simulink model "Protection"  (R2023b)
settings: Solver=FixedStepAuto  StartTime=0.0  StopTime=2  RelTol=1e-3
InitFcn:
  | Ts_Control=100e-6;
  | fs=50000;
  | Ts=1/fs/10;
  | Ts_Power=Ts;
  | Ts_control=5*Ts;
  | wnom=314.16;
  | Lf=5e-3;
  | Rf=0.1;
  | Cf=50e-6;
  | 
  | 
  | % choosing crossover frequency
  | fc=(1/10)*fs;
  | wc=2*pi*fc;
  | Ti=1/wc;
  | Kpc=Lf/Ti;
  | 
  | Kic=Rf/Ti;
  | 
  | x=[837.555 8.2389 0.057896 268.1361 0.74685 242.918 0.062838 291.0935]
  | 
  | 
  | Kvi=x(1);Kvp=x(2);Kcp=x(3);Kci=x(4);
  | Kvpb=x(5);Kvib=x(6);Kcpb=x(7);Kcib=x(8);
  | 
  | 
  | x1=[0.202905850069502  0.158544693742674   0.10408       75.97091  837.555350377473 8.2389271001531  0.10408       75.97091];
  | 
  | Kvif=x1(1);Kvpf=x1(2);Kcpf=x1(3);Kcif=x1(4);
  | Kvim=x1(5);Kvpm=x1(6);Kcpm=x1(7);Kcim=x1(8);
undefined symbols (not defined in the file): D1, Delta, Hydride, Metal, Nickel, sigbuilder_block
libraries: spsSeriesRLCBranchLib x52, spsVoltageMeasurementLib x22, powerlib_extras x18, spsCurrentMeasurementLib x13, spsIdealSwitchLib x12, simulink x8, slpidlib x7, spsGroundLib x6, spsBreakerLib x5, spsDiodeLib x4, spsIGBTLib x4, spsThreePhaseVIMeasurementLib x4
(part 1 of 2)
settings Model: Creator=shiva  LastModifiedBy=vnougain
settings SolverCC: AlgebraicLoopSolver=TrustRegion
settings DataIOCC: LimitDataPoints=on  SaveOutput=off  SaveTime=off  ReturnWorkspaceOutputs=off
settings OptimizationCC: EfficientMapNaN2IntZero=off  LifeSpan=inf
settings DebuggingCC: UnconnectedInputMsg=warning  UnconnectedOutputMsg=warning  UnconnectedLineMsg=warning  AllowSymbolicDim=off  SFUnexpectedBacktrackingDiag=warning  SFNoUnconditionalDefaultTransitionDiag=warning  SFExecutionAtInitializationDiag=none  ArithmeticOperatorsInVariantConditions=warning
settings HardwareCC: ProdBitPerChar=16  ProdBitPerInt=16  ProdBitPerPointer=32  ProdBitPerSizeT=32  ProdBitPerPtrDiffT=32  ProdLargestAtomicInteger=Integer  ProdLargestAtomicFloat=None  ProdWordSize=16  ProdHWDeviceType=Texas Instruments->C2000  TargetBitPerPointer=64  TargetBitPerSizeT=64  TargetBitPerPtrDiffT=64  TargetLongLongMode=on  TargetIntDivRoundTo=Zero  TargetEndianess=LittleEndian  TargetWordSize=64  TargetHWDeviceType=MATLAB Host  ProdEqTarget=off
settings ModelReferenceCC: EnableRefExpFcnMdlSchedulingChecks=on  PropagateSignalLabelsOutOfModel=off
settings SFSimCC: SimUseLocalCustomCode=off  CustomCodeUndefinedFunction=UseInterfaceOnly
settings RTWCC: RTWUseLocalCustomCode=off
settings CodeAppCC: MaxIdLength=128  StateflowObjectComments=on
settings GRTTargetCC: TargetLangStandard=C89/C90 (ANSI)  CombineOutputUpdateFcns=off  GRTInterface=on
settings ConfigComp: CovMetricSettings=dw  CovSaveCumulativeToWorkspaceVar=on  CovSaveSingleToWorkspaceVar=on  CovExternalEMLEnable=off
settings SimscapeCC: SimscapeNormalizeSystem=off
settings TargetHardwareResources: Description=Target Hardware Resources Component

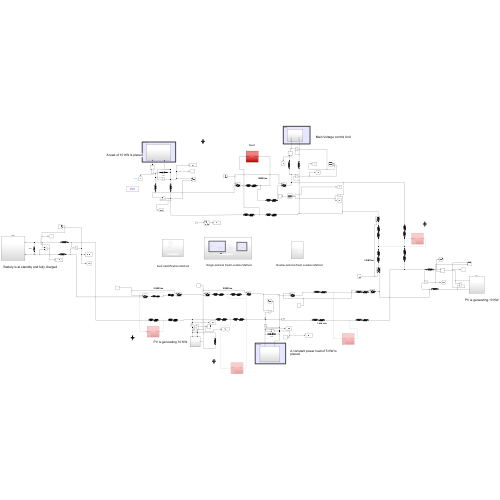
[thumbnail: Simulink's stored preview of the top-level diagram]
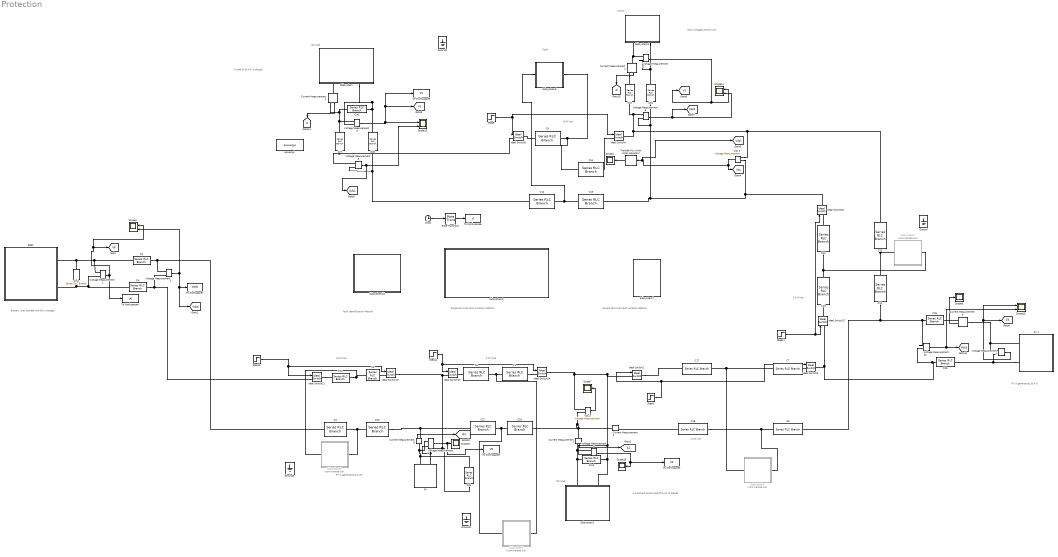
== system Protection ==
  note: Utility
  note: DC load
  note: DC load
  note: 2KM line
  note: 3 KM line
  note: 2 KM line
  note: 1 KM line
  note: 3 KM line
  note: A load of 10 KW is placed
  note: A constant power load of 5 KW is placed
  note: PV is generating 10 KW
  note: Battery is at standby and fully charged
  note: Main Voltage control Unit
  note: Fault
  note: Single-terminal Fault Location Method
  note: Double-terminal Fault Location Method
  note: PV is generating 10 KW
  note: Fault Identification Method
  C{1,6,19,22} (4 alike) : spsSeriesRLCBranchLib/Series RLC Branch  LConnTagsString=__new0  RConnTagsString=__new0  BranchType=RL  Resistance=1*0.3293  Inductance=1*522.026e-6  SetiL0=off  InitialCurrent=0  Capacitance=12000e-06  Setx0=off  InitialVoltage=0  Measurements=None
  C{9..12,23..24} (6 alike) : spsSeriesRLCBranchLib/Series RLC Branch  LConnTagsString=__new0  RConnTagsString=__new0  BranchType=RL  Resistance=0.3293*1.5  Inductance=522.026e-6*1.5  SetiL0=off  InitialCurrent=0  Capacitance=12000e-06  Setx0=off  InitialVoltage=0  Measurements=None
  C13 : spsSeriesRLCBranchLib/Series RLC Branch  LConnTagsString=__new0  RConnTagsString=__new0  BranchType=RL  Resistance=0.3293*0.5  Inductance=522.026e-6*0.5  SetiL0=off  InitialCurrent=0  Capacitance=12000e-06  Setx0=off  InitialVoltage=0  Measurements=None
  C14 : spsSeriesRLCBranchLib/Series RLC Branch  LConnTagsString=__new0  RConnTagsString=__new0  BranchType=RL  Resistance=0.3293*0.5  Inductance=522.026e-6*0.5  SetiL0=off  InitialCurrent=0  Capacitance=12000e-06  Setx0=off  InitialVoltage=0  Measurements=None
  C{15..16,27..28} (4 alike) : spsSeriesRLCBranchLib/Series RLC Branch  LConnTagsString=__new0  RConnTagsString=__new0  BranchType=L  Resistance=1.5*0.3293  Inductance=1e-3  SetiL0=off  InitialCurrent=0  Capacitance=12000e-06  Setx0=off  InitialVoltage=0  Measurements=None
  C{7..8,17..18} (4 alike) : spsSeriesRLCBranchLib/Series RLC Branch  LConnTagsString=__new0  RConnTagsString=__new0  BranchType=RL  Resistance=0.3293/2  Inductance=(522.026e-6)/2  SetiL0=off  InitialCurrent=0  Capacitance=12000e-06  Setx0=off  InitialVoltage=0  Measurements=None
  C2 : spsSeriesRLCBranchLib/Series RLC Branch  LConnTagsString=__new0  RConnTagsString=__new0  BranchType=L  Resistance=1.5*0.3293  Inductance=5e-6  SetiL0=off  InitialCurrent=0  Capacitance=12000e-06  Setx0=off  InitialVoltage=0  Measurements=None
  C{3,5,20..21} (4 alike) : spsSeriesRLCBranchLib/Series RLC Branch  LConnTagsString=__new0  RConnTagsString=__new0  BranchType=RL  Resistance=1.5*0.3293  Inductance=1.5*522.026e-6  SetiL0=off  InitialCurrent=0  Capacitance=12000e-06  Setx0=off  InitialVoltage=0  Measurements=None
  C25 : spsSeriesRLCBranchLib/Series RLC Branch  LConnTagsString=__new0  RConnTagsString=__new0  BranchType=R  Resistance=245  Inductance=1*522.026e-6  SetiL0=off  InitialCurrent=0  Capacitance=12000e-06  Setx0=off  InitialVoltage=0  Measurements=None
  C26 : spsSeriesRLCBranchLib/Series RLC Branch  LConnTagsString=__new0  RConnTagsString=__new0  BranchType=L  Resistance=1.5*0.3293  Inductance=5e-9  SetiL0=off  InitialCurrent=0  Capacitance=12000e-06  Setx0=off  InitialVoltage=0  Measurements=None
  C29 : spsSeriesRLCBranchLib/Series RLC Branch  LConnTagsString=__new0  RConnTagsString=__new0  BranchType=L  Resistance=1.5*0.3293  Inductance=5e-9  SetiL0=off  InitialCurrent=0  Capacitance=12000e-06  Setx0=off  InitialVoltage=0  Measurements=None
  C4 : spsSeriesRLCBranchLib/Series RLC Branch  LConnTagsString=__new0  RConnTagsString=__new0  BranchType=L  Resistance=1.5*0.3293  Inductance=5e-6  SetiL0=off  InitialCurrent=0  Capacitance=12000e-06  Setx0=off  InitialVoltage=0  Measurements=None
  Cin1 : spsSeriesRLCBranchLib/Series RLC Branch  LConnTagsString=__new0  RConnTagsString=__new0  BranchType=C  Resistance=1  Inductance=1e-3  SetiL0=off  InitialCurrent=0  Capacitance=5000e-6  Setx0=on  InitialVoltage=700  Measurements=None
  Cin2 : spsSeriesRLCBranchLib/Series RLC Branch  LConnTagsString=__new0  RConnTagsString=__new0  BranchType=C  Resistance=1  Inductance=1e-3  SetiL0=off  InitialCurrent=0  Capacitance=1000e-6  Setx0=on  InitialVoltage=700  Measurements=None
  Cin4 : spsSeriesRLCBranchLib/Series RLC Branch  LConnTagsString=__new0  RConnTagsString=__new0  BranchType=C  Resistance=1  Inductance=1e-3  SetiL0=off  InitialCurrent=0  Capacitance=1000e-6  Setx0=on  InitialVoltage=700  Measurements=None
  Clock : Clock
      settings: Decimation=6
  Current Measurement{1..2,4..7} (6 alike) : spsCurrentMeasurementLib/Current Measurement  PhasorSimulation=off  OutputType=Complex  PSBequivalent=0
  ESS1 : Subsystem
  Ground{,1,3..4} (4 alike) : spsGroundLib/Ground  LConnTagsString=a
  Ideal Switch{4..5,10..11,13..14,16..17} (8 alike) : spsIdealSwitchLib/Ideal Switch  Ron=1  Lon=0  IC=0  Rs=1e5  Cs=inf  Measurements=off
  Ideal Switch2 : spsIdealSwitchLib/Ideal Switch  Ron=0.00001  Lon=0  IC=0  Rs=1e5  Cs=inf  Measurements=off
  Ideal Switch3 : spsIdealSwitchLib/Ideal Switch  Ron=0.00001  Lon=0  IC=0  Rs=1e5  Cs=inf  Measurements=off
  "PV " : Subsystem
  PV 1 : Subsystem
  Rate Transition : RateTransition  OutPortSampleTime=Ts
  Scope{2,13..15} (4 alike) : Scope  NumInputPorts=2
  Scope{3..4,7,16..17} (5 alike) : Scope
  Step11 : Step  Time=10  Before=1  After=0  SampleTime=0
  Step14 : Step  Time=10  Before=1  After=0  SampleTime=0
  Step17 : Step  Time=1.041  Before=1  After=0  SampleTime=0
  Step4 : Step  Time=10  Before=1  SampleTime=0
  Step5 : Step  Time=10  Before=1  After=0  SampleTime=0
  Subsystem : Subsystem
  Subsystem1 : Subsystem
  Subsystem10 : Subsystem
  Subsystem2 : Subsystem  Commented=on
  Subsystem3 : Subsystem  Commented=on
  Subsystem4 : Subsystem
  Subsystem5 : Subsystem  Commented=on
  Subsystem6 : Subsystem
  Subsystem7 : Subsystem
  Subsystem8 : Subsystem  Commented=on
  Subsystem9 : Subsystem
  To Workspace1 : ToWorkspace  VariableName=V4  SaveFormat=Structure With Time  SampleTime=-1
      settings: Decimation=6
  To Workspace3 : ToWorkspace  VariableName=V5  SaveFormat=Structure With Time  SampleTime=-1
      settings: Decimation=6
  To Workspace4 : ToWorkspace  VariableName=V6  SaveFormat=Structure With Time  SampleTime=-1
      settings: Decimation=6
  To Workspace5 : ToWorkspace  VariableName=V1  SaveFormat=Structure With Time  SampleTime=-1
      settings: Decimation=6
  To Workspace6 : ToWorkspace  VariableName=d  SaveFormat=Structure With Time  SampleTime=-1
      settings: Decimation=6
  To Workspace7 : ToWorkspace  VariableName=Vdc6  SaveFormat=Structure With Time  SampleTime=-1
      settings: Decimation=6
  Transfer Fcn (with initial outputs)2 : simulink_extras/Additional Linear/Transfer Fcn (with initial outputs)  N=[5*31.416]  D="[1  5*31.416]"  Y0=700  U0=700
  Vdc 2 : spsVoltageMeasurementLib/Voltage Measurement  Tag=PoWeRsYsTeMmEaSuReMeNt  PhasorSimulation=off  OutputType=Magnitude  PSBequivalent=0
  Vdc 3 : spsVoltageMeasurementLib/Voltage Measurement  Tag=PoWeRsYsTeMmEaSuReMeNt  PhasorSimulation=off  OutputType=Magnitude  PSBequivalent=0
  Voltage Measurement{1..10} (10 alike) : spsVoltageMeasurementLib/Voltage Measurement  PhasorSimulation=off  OutputType=Complex  PSBequivalent=0
  powergui : sps_lib/powergui  Priority=1  SimulationMode=Discrete  SampleTime=Ts  frequency=60  Iterations=50  frequencyindice=0  Pbase=100e6  ErrMax=1e-4  UnitsV=kV  UnitsW=MW  buscounter=0  FunctionMessages=off  echomessages=off  EnableUseOfTLC=off  CurrentSourceSwitches=off  DisableSnubberDevices=off  DisableRonSwitches=off  DisableVfSwitches=off  DisplayEquations=off  AutomaticDiscreteSolvers=off  SolverType=Tustin/Backward Euler (TBE)  Interpol=off  ExternalGateDelay=off  methode=off  Ts=0  x0status=blocks  SPID=off  SwTol=0  HookPort=off  NonlinearTolerance=1e-4  nMaxIteration=100  ContinueOnMaxIteration=off  RestoreLinks=warning  ResistiveCurrentMeasurement=off  Frange=[0:2:500]  Ylog=off  Xlog=on  ShowGrid=off  save=off  variable=ZData  structure=SR1  ZoomFFT=off  StartTime=3.4  cycles=10  DisplayStyle=1  fundamental=15  FreqAxis=off  MaxFrequency=100  frequencyindicesteady=1  RmsSteady=1  display=off
  tag scope: IL2=global, IPV=global, Udc1=global, V1=global, V2=global, V3=global, V6=global, Vdc1=global, Vdc2=global, Vdc3=global, Vdc6=global, Vdc=global, i1=global, i2=global
  wires:
  Current Measurement5/1 -> Scope3/1
  Vdc 2/1 -> Scope7/1
  Vdc 3/1 -> [Vdc1], Transfer Fcn (with initial outputs)2/1, [Vdc]
  Voltage Measurement1/1 -> Scope2/1, [V6], To Workspace4/1
  Current Measurement6/1 -> [IPV]
  Current Measurement7/1 -> [IL2]
  Step4/1 -> Ideal Switch2/1, Ideal Switch3/1
  Step5/1 -> Ideal Switch4/1, Ideal Switch5/1
  Step11/1 -> Ideal Switch11/1, Ideal Switch10/1
  Step14/1 -> Ideal Switch14/1, Ideal Switch13/1
  Step17/1 -> Ideal Switch17/1, Ideal Switch16/1
  Transfer Fcn (with initial outputs)2/1 -> Scope4/1
  Voltage Measurement3/1 -> To Workspace5/1, [V1], Scope13/1
  Voltage Measurement2/1 -> [V2], Scope14/1
  Voltage Measurement4/1 -> [V3], Scope15/1
  Voltage Measurement5/1 -> Scope16/1, To Workspace1/1
  Voltage Measurement6/1 -> To Workspace3/1, Scope17/1
  Clock/1 -> Rate Transition/1
  Rate Transition/1 -> To Workspace6/1
  Voltage Measurement7/1 -> [Vdc6], To Workspace7/1, Scope2/2
  Voltage Measurement8/1 -> Scope13/2, [Udc1]
  Voltage Measurement9/1 -> [Vdc2], Scope14/2
  Voltage Measurement10/1 -> Scope15/2, [Vdc3]
  Current Measurement1/1 -> [i1]
  Current Measurement2/1 -> [i2]
  connections:
  C8/LConn1 -- C26/RConn1 -- Voltage Measurement10/LConn1 -- C11/RConn1
  C20/LConn1 -- Current Measurement6/RConn1 -- C22/RConn1
  C3/RConn1 -- Voltage Measurement7/LConn1 -- C2/LConn1
  C1/RConn1 -- Subsystem2/RConn1 -- C6/LConn1
  Cin1/RConn1 -- C28/RConn1 -- Voltage Measurement3/LConn2 -- Subsystem/RConn2
  C4/LConn1 -- Voltage Measurement7/LConn2 -- Ideal Switch11/LConn1
  Voltage Measurement6/LConn2 -- "PV "/RConn2 -- C25/LConn1 -- Ideal Switch10/RConn1 -- Ideal Switch13/LConn1
  Current Measurement4/LConn1 -- Current Measurement7/LConn1 -- C19/LConn1 -- Vdc 2/LConn1
  C13/RConn1 -- Subsystem6/LConn1 -- C12/LConn1
  Current Measurement5/LConn1 -- Voltage Measurement4/LConn1 -- PV 1/RConn1
  C9/LConn1 -- Subsystem6/RConn1 -- C14/RConn1
  C24/RConn1 -- Subsystem5/RConn1 -- C10/LConn1
  C7/RConn1 -- Subsystem3/LConn1 -- C17/LConn1
  C18/LConn1 -- Subsystem3/RConn1 -- C8/RConn1
  Cin4/LConn1 -- Voltage Measurement5/LConn1 -- Current Measurement7/RConn1 -- Subsystem1/RConn1
  PV 1/RConn2 -- C29/LConn1 -- Voltage Measurement4/LConn2
  Voltage Measurement2/LConn1 -- Current Measurement2/LConn1 -- Subsystem4/LConn1
  C18/RConn1 -- Current Measurement4/RConn1
  Ideal Switch2/RConn1 -- C17/RConn1
  C7/LConn1 -- Ideal Switch3/LConn1
  Ideal Switch4/LConn1 -- C14/LConn1
  C9/RConn1 -- Ideal Switch5/RConn1
  C20/RConn1 -- Subsystem8/RConn1 -- C3/LConn1
  C21/LConn1 -- Subsystem8/LConn1 -- C5/RConn1
  Ideal Switch10/LConn1 -- C5/LConn1
  Ideal Switch11/RConn1 -- C21/RConn1
  Subsystem1/RConn2 -- Cin4/RConn1 -- Voltage Measurement5/LConn2 -- Ideal Switch2/LConn1 -- Ideal Switch14/RConn1 -- Vdc 2/LConn2
  Ideal Switch13/RConn1 -- C6/RConn1
  C1/LConn1 -- Ideal Switch14/LConn1
  C11/LConn1 -- Subsystem5/LConn1 -- C23/RConn1
  C24/LConn1 -- Ideal Switch16/LConn1
  Ideal Switch17/RConn1 -- C10/RConn1
  "PV "/RConn1 -- C25/RConn1 -- Voltage Measurement6/LConn1 -- Current Measurement6/LConn1
  C19/RConn1 -- Subsystem2/LConn1 -- C22/LConn1
  C2/RConn1 -- Cin2/LConn1 -- ESS1/RConn1 -- Voltage Measurement1/LConn1
  Cin2/RConn1 -- Voltage Measurement1/LConn2 -- C4/RConn1 -- ESS1/RConn2
  C27/RConn1 -- Voltage Measurement3/LConn1 -- Current Measurement1/RConn1 -- Cin1/LConn1
  Vdc 3/LConn1 -- C15/LConn1 -- Voltage Measurement9/LConn1 -- Ideal Switch4/RConn1 -- C23/LConn1
  Subsystem4/LConn2 -- C16/RConn1 -- Voltage Measurement2/LConn2
  Current Measurement5/RConn1 -- C26/LConn1
  Voltage Measurement10/LConn2 -- Ideal Switch3/RConn1 -- Ideal Switch17/LConn1 -- C29/RConn1
  Current Measurement1/LConn1 -- Subsystem/RConn1
  Current Measurement2/RConn1 -- C15/RConn1
  Vdc 3/LConn2 -- C13/LConn1 -- C16/LConn1 -- Voltage Measurement9/LConn2 -- Ideal Switch16/RConn1
  C27/LConn1 -- Voltage Measurement8/LConn1 -- Ideal Switch5/LConn1
  C28/LConn1 -- Voltage Measurement8/LConn2 -- C12/RConn1

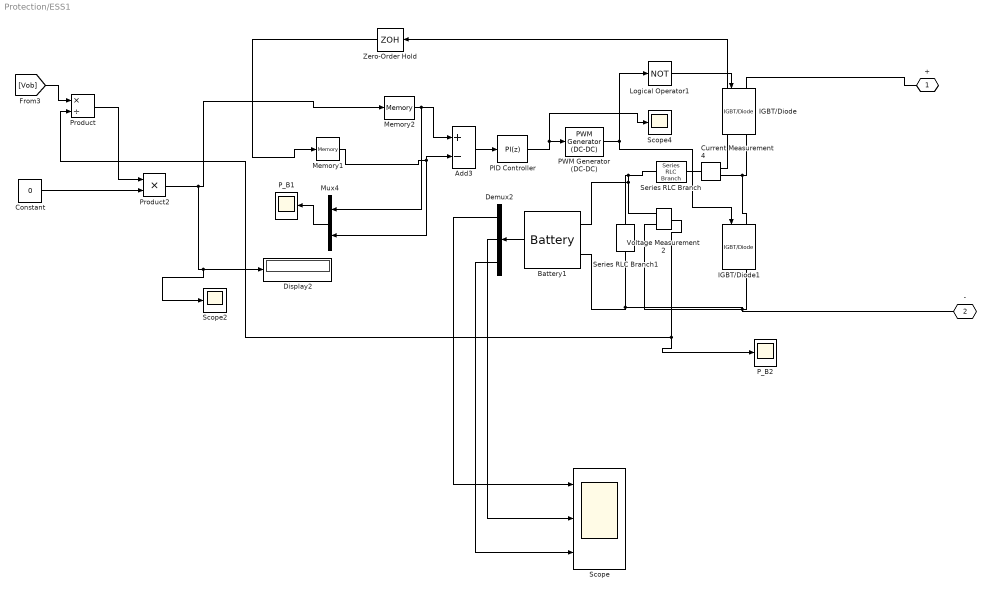
== system Protection/ESS1 ==
  Add3 : Sum  Inputs=+-
  Battery1 : spsBatteryLib/Battery  BatType=Nickel-Metal-Hydride  ShowTempParam=off  ThermalPreset=no  ShowAgeParam=off  NomV=300  NomQ=200  SOC=100  Batt_Tr=30  PresetModel=on  MaxQ=215.3846  MinV=225  FullV=353.3898  Dis_rate=40  R=0.015  Normal_OP=192.3077  expZone="[325.4237            40]"  current=[6.5 13 32.5]  Units=Time  Tci=20  NomT=20  T2=-30  MaxQ2=4.8  FullV2=7.1  Normal_OP2=5.72  expZone2="[6.58  1]"  Rca=0.6  ti=1000  Dp=0  Neq0=0  Tsim=1e6  Ta1=25  Qeol=5.4*0.9  Reol=0.013333*1.2  Char_age=[2.3478, 3]  Dis_age=[2.3478, 10]  N1=1500  N2=10500  N3=1000  N4=1400  Ta2=45  N5=950
      settings: LibrarySourceBlock=electricdrivelib/Extra Sources/Battery
  Constant : Constant  Value=0
  Current Measurement4 : spsCurrentMeasurementLib/Current Measurement  PhasorSimulation=off  OutputType=Complex  PSBequivalent=0
  Demux2 : Demux  Outputs=3
  Display2 : Display
  IGBT/Diode : spsIGBTDiodeLib/IGBT//Diode  Ron=1e-3  Rs=1e5  Cs=inf  Measurements=on
  IGBT/Diode1 : spsIGBTDiodeLib/IGBT//Diode  Ron=1e-3  Rs=1e5  Cs=inf  Measurements=on
  Logical Operator1 : Logic  Operator=NOT  AllPortsSameDT=off  OutDataTypeStr=boolean
  Memory1 : Memory
  Memory2 : Memory
  Mux4 : Mux  Inputs=2
  PID Controller : slpidlib/PID Controller  Controller=PI  Form=Parallel  TimeDomain=Discrete-time  UseExternalTs=off  SampleTime=Ts_Control  IntegratorMethod=Forward Euler  FilterMethod=Forward Euler  ControllerParametersSource=internal  P=0.03  I=50  UseKiTs=off  D=0  N=100  UseFilter=on  TunerSelectOption=Transfer Function Based (PID Tuner App)  InitialConditionSource=internal  InitialConditionForIntegrator=0  InitialConditionForFilter=0  DifferentiatorICPrevScaledInput=0  ExternalReset=none  TrackingMode=off  Kt=1  LimitOutput=on  SatLimitsSource=internal  UpperSaturationLimit=1  LowerSaturationLimit=0  LinearizeAsGain=on  AntiWindupMode=none  Kb=1  LimitIntegrator=off  UpperIntegratorSaturationLimit=inf  LowerIntegratorSaturationLimit=-inf  POutMin=[]  POutMax=[]  IOutMin=[]  IOutMax=[]  DOutMin=[]  DOutMax=[]  NOutMin=[]  NOutMax=[]  SumOutMin=[]  SumOutMax=[]  SaturationOutMin=[]  SaturationOutMax=[]  PParamMin=[]  PParamMax=[]  IParamMin=[]  IParamMax=[]  DParamMin=[]  DParamMax=[]  NParamMin=[]  NParamMax=[]  KbParamMin=[]  KbParamMax=[]  KtParamMin=[]  KtParamMax=[]  KbOutMin=[]  KbOutMax=[]  KtOutMin=[]  KtOutMax=[]  IntegratorOutMin=[]  IntegratorOutMax=[]  FilterOutMin=[]  FilterOutMax=[]  SumI1OutMin=[]  SumI1OutMax=[]  SumI2OutMin=[]  SumI2OutMax=[]  SumI3OutMin=[]  SumI3OutMax=[]  SumI4OutMin=[]  SumI4OutMax=[]  SumDOutMin=[]  SumDOutMax=[]  DifferentiatorOutMin=[]  DifferentiatorOutMax=[]  FilterDiffOutCoefMin=[]  FilterDiffOutCoefMax=[]  ReciprocalOutMin=[]  ReciprocalOutMax=[]  SumDenOutMin=[]  SumDenOutMax=[]  SumNumOutMin=[]  SumNumOutMax=[]  DivideOutMin=[]  DivideOutMax=[]  UdiffTsProdOutMin=[]  UdiffTsProdOutMax=[]  NTsProdOutMin=[]  NTsProdOutMax=[]  UintegralTsProdOutMin=[]  UintegralTsProdOutMax=[]  UngainTsProdOutMin=[]  UngainTsProdOutMax=[]  ClampingZeroOutDataTypeStr=Inherit: Inherit via back propagation  ClampingZeroOutMin=[]  ClampingZeroOutMax=[]  FilterDenConstantOutDataTypeStr=Inherit: Inherit via back propagation  FilterDenConstantOutMin=[]  FilterDenConstantOutMax=[]  PCopyOutDataTypeStr=Inherit: Inherit via back propagation  PCopyOutMin=[]  PCopyOutMax=[]  NCopyOutDataTypeStr=Inherit: Inherit via back propagation  NCopyOutMin=[]  NCopyOutMax=[]  IntegratorContinuousStateAttributes=''  IntegratorStateMustResolveToSignalObject=off  IntegratorRTWStateStorageClass=Auto  FilterContinuousStateAttributes=''  FilterStateMustResolveToSignalObject=off  FilterRTWStateStorageClass=Auto  ParallelPVariant=InternalParameters  IdealPVariant=Disabled  IVariant=InternalParameters  DVariant=Disabled  IntegratorVariant=Discrete  SatVariant=Enabled  AWVariant=Passthrough  PCopyVariant=Disabled  TRVariant=Disabled  FdbkBlocksVariant=Forward  IdealPFdbkVariant=Disabled  SatFdbkVariant=Disabled  DerivativeFilterVariant=Disabled  NVariant=Disabled  NCopyVariant=Disabled_SignalSpec  FilterICVariant=Disabled  IntegratorICVariant=InternalICs  ExternalResetVariant=Disabled  TRSumVariant=Passthrough  SumFdbkVariant=Disabled  SumVariant=Sum_PI  TsampFilterVariant=InternalTs  TsampNgainVariant=Passthrough  TsampIntegralVariant=Disabled_SignalSpec  ExternalSaturationOutDataTypeStr=Inherit: Same as second input
  PWM Generator (DC-DC) : spsPWMGeneratorDCDCLib/PWM Generator (DC-DC)  Fsw=10000  Ts=Ts
  P_B1 : Scope
  P_B2 : Scope
  Product : Product  Inputs=*/
  Product2 : Product  Inputs=**
  Scope : Scope  NumInputPorts=3
  Scope2 : Scope
  Scope4 : Scope
  Series RLC Branch : spsSeriesRLCBranchLib/Series RLC Branch  LConnTagsString=__new0  RConnTagsString=__new0  BranchType=RL  Resistance=0.1  Inductance=9.2e-3  SetiL0=on  InitialCurrent=0  Capacitance=1e-6  Setx0=off  InitialVoltage=0  Measurements=None
  Series RLC Branch1 : spsSeriesRLCBranchLib/Series RLC Branch  LConnTagsString=__new0  RConnTagsString=__new0  BranchType=C  Resistance=1  Inductance=1e-3  SetiL0=off  InitialCurrent=0  Capacitance=1000e-6  Setx0=on  InitialVoltage=354  Measurements=None
  Voltage Measurement2 : spsVoltageMeasurementLib/Voltage Measurement  PhasorSimulation=off  OutputType=Complex  PSBequivalent=0
  Zero-Order Hold : ZeroOrderHold  SampleTime=Ts
  + : PMIOPort  Tag=PMCPort  Side=Right
  - : PMIOPort  Tag=PMCPort  Port=2  Side=Right
  wires:
  Battery1/1 -> Demux2/1
  Mux4/1 -> P_B1/1
  Zero-Order Hold/1 -> Memory1/1
  Logical Operator1/1 -> IGBT/Diode/1
  Current Measurement4/1 -> Zero-Order Hold/1
  Demux2/1 -> Scope/1
  Demux2/2 -> Scope/2
  Demux2/3 -> Scope/3
  Add3/1 -> PID Controller/1
  PWM Generator (DC-DC)/1 -> IGBT/Diode1/1, Logical Operator1/1
  Memory2/1 -> Mux4/1, Add3/1
  Voltage Measurement2/1 -> Product/2, P_B2/1
  Product2/1 -> Scope2/1, Display2/1, Memory2/1
  Memory1/1 -> Mux4/2, Add3/2
  PID Controller/1 -> Scope4/1, PWM Generator (DC-DC)/1
  [Vob] -> Product/1
  Product/1 -> Product2/1
  Constant/1 -> Product2/2
  connections:
  Series RLC Branch1/LConn1 -- Series RLC Branch/LConn1 -- Battery1/LConn1 -- Voltage Measurement2/LConn1
  IGBT/Diode/RConn1 -- Current Measurement4/RConn1 -- IGBT/Diode1/LConn1
  Voltage Measurement2/LConn2 -- -/RConn1 -- Series RLC Branch1/RConn1 -- Battery1/LConn2 -- IGBT/Diode1/RConn1
  Series RLC Branch/RConn1 -- Current Measurement4/LConn1
  IGBT/Diode/LConn1 -- +/RConn1

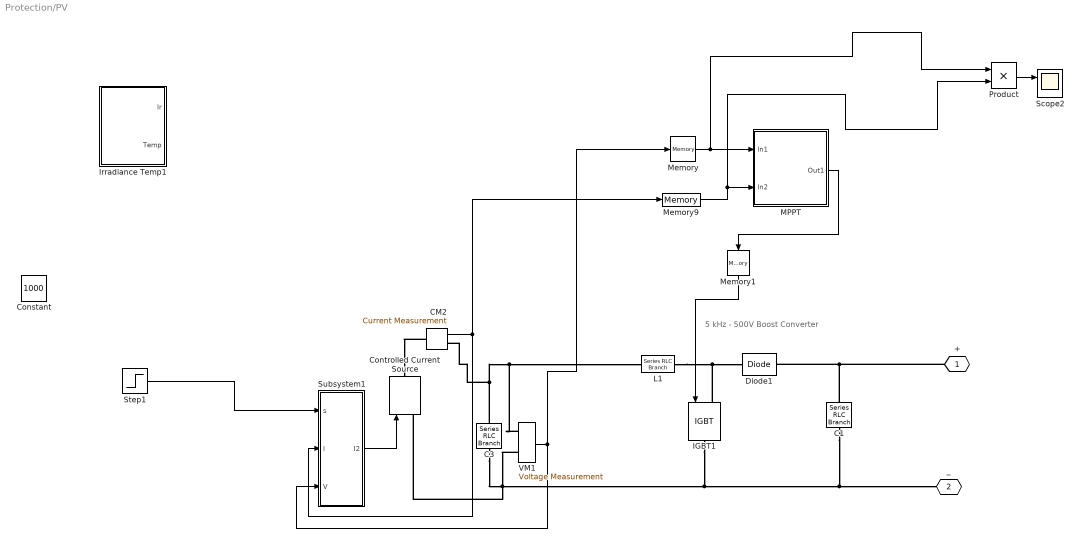
== system Protection/PV  ==
  note: 5 kHz - 500V
      | Boost Converter
  C1 : spsSeriesRLCBranchLib/Series RLC Branch  LConnTagsString=__new0  RConnTagsString=__new0  BranchType=C  Resistance=1.0  Inductance=1.0  SetiL0=off  InitialCurrent=0  Capacitance=1000e-6  Setx0=on  InitialVoltage=700  Measurements=Branch voltage
  C3 : spsSeriesRLCBranchLib/Series RLC Branch  LConnTagsString=__new0  RConnTagsString=__new0  BranchType=C  Resistance=1.0  Inductance=1.0  SetiL0=off  InitialCurrent=0  Capacitance=100e-6  Setx0=on  InitialVoltage=250  Measurements=Branch voltage
  CM2 : spsCurrentMeasurementLib/Current Measurement  Tag=PoWeRsYsTeMmEaSuReMeNt  PhasorSimulation=off  OutputType=Magnitude  PSBequivalent=0
      settings: AttributesFormatString=\n
  Constant : Constant  Value=1000
  Controlled Current Source : spsControlledCurrentSourceLib/Controlled Current Source  Initialize=off  Source_Type=DC  Amplitude=0  Phase=0  Frequency=0  Measurements=None
  Diode1 : spsDiodeLib/Diode  Ron=1e-4  Lon=0  Vf=0  IC=0  UseSnubber=off  Rs=inf  Cs=inf  Measurements=off
  IGBT1 : spsIGBTLib/IGBT  Ron=0.001  Lon=0  Vf=0  Tf=0  Tt=0  IC=0  Rs=1e5  Cs=inf  Measurements=off
  Irradiance Temp1 : Subsystem  Tag=STV Subsys  LoadFcn=sigbuilder_block('load');  StartFcn=sigbuilder_block('start');  StopFcn=sigbuilder_block('stop');  ClipboardFcn=sigbuilder_block('clipboard');  mask(Sigbuilder block){tuvar=[0:10]}
      mask help: Sigbuilder GUI
      mask init:
      | if ~strcmp(get_param(bdroot(gcbh),'SimulationStatus'),'stopped') tuvar = sigbuilder_block('maskInit'); end
      settings: CopyFcn=sigbuilder_block('copy');  DeleteFcn=sigbuilder_block('delete');  ModelCloseFcn=sigbuilder_block('modelClose');  PreSaveFcn=sigbuilder_block('preSave');  PauseFcn=sigbuilder_block('pause')  ContinueFcn=sigbuilder_block('continue')  NameChangeFcn=sigbuilder_block('namechange');  OpenFcn=sigbuilder_block('open',[216.75 153.75 550.5 395.25 ]);  CloseFcn=sigbuilder_block('close');
      mask Display: plot(0, 0, 100, 100,[2, 2, 32, 32, 2], [68, 8, 8, 68, 68],[32, 2], [38, 38], [32, 19, 2],[53, 60, 44], [32, 17, 17, 2],[16, 16, 31, 31]);txt = getActiveGroup(gcbh);text(2, 100, txt,'verticalAlignment', 'top');
  L1 : spsSeriesRLCBranchLib/Series RLC Branch  LConnTagsString=__new0  RConnTagsString=__new0  BranchType=RL  Resistance=0.005  Inductance=5e-3  SetiL0=off  InitialCurrent=0  Capacitance=1e-6  Setx0=off  InitialVoltage=0  Measurements=None
  MPPT : Subsystem
  Memory : Memory  InheritSampleTime=on
  Memory1 : Memory  InheritSampleTime=on
  Memory9 : Memory  InheritSampleTime=on
  Product : Product
  Scope2 : Scope  NumInputPorts=2
  Step1 : Step  Time=5  Before=1000  After=1000  SampleTime=0
  Subsystem1 : Subsystem  mask{A=1.9, T=315, s=1000, Rs=0.01, Rp=400, ns=600, np=3}
      mask prompts: A "Ideality Factor"; T "Surface Temp(K)"; s "Solar Irradiance(W/m^2)"; Rs "Series Resistance"; Rp "Parallel Resistance"; ns "No. of series cell"; np "No. of parallel cell"
      mask init:
      | k=1.38e-23;
      | Voc_n=32.9;
      | Isc_n=10.21;
      | Ki=3.18e-3;
      | Tr=301.15;
      | q=1.6e-19;
      | Eg=1.1;
      | s_n=1000;
  VM1 : spsVoltageMeasurementLib/Voltage Measurement  Tag=PoWeRsYsTeMmEaSuReMeNt  PhasorSimulation=off  OutputType=Magnitude  PSBequivalent=0
  + : PMIOPort  Tag=PMCPort  Side=Right
  _ : PMIOPort  Tag=PMCPort  Port=2  Side=Right
  wires:
  Subsystem1/1(I2) -> Controlled Current Source/1
  CM2/1 -> Subsystem1/2(I), Memory9/1
  VM1/1 -> Subsystem1/3(V), Memory/1
  Memory/1 -> Product/1, MPPT/1(In1)
  Memory9/1 -> Product/2, MPPT/2(In2)
  MPPT/1(Out1) -> Memory1/1
  Memory1/1 -> IGBT1/1
  Product/1 -> Scope2/1
  Step1/1 -> Subsystem1/1(s)
  connections:
  +/RConn1 -- C1/LConn1 -- Diode1/RConn1
  L1/RConn1 -- IGBT1/LConn1 -- Diode1/LConn1
  VM1/LConn2 -- Controlled Current Source/LConn1 -- C3/RConn1 -- IGBT1/RConn1 -- C1/RConn1 -- _/RConn1
  C3/LConn1 -- CM2/RConn1 -- VM1/LConn1 -- L1/LConn1
  CM2/LConn1 -- Controlled Current Source/RConn1

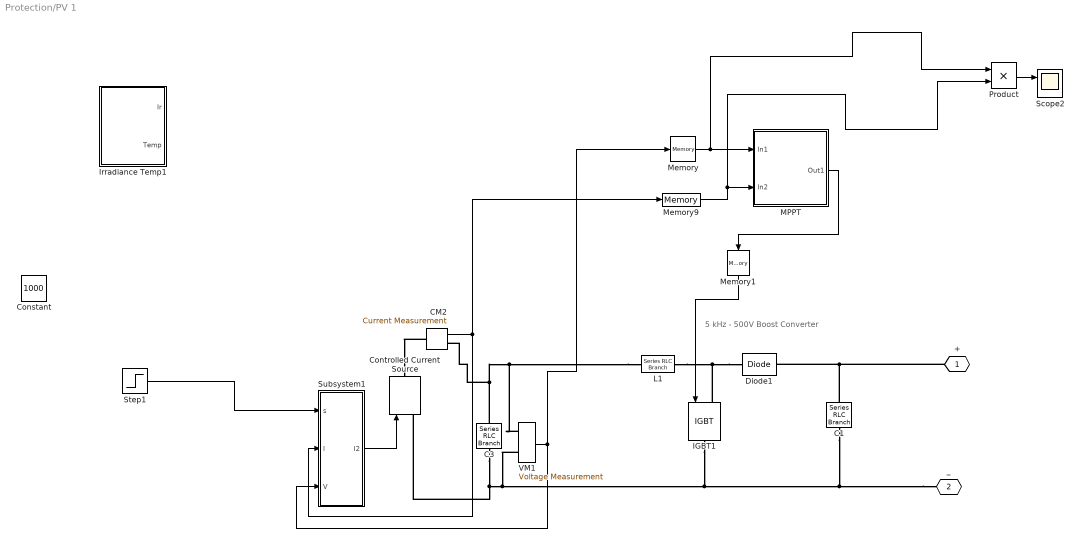
== system Protection/PV 1 ==
  note: 5 kHz - 500V
      | Boost Converter
  C1 : spsSeriesRLCBranchLib/Series RLC Branch  LConnTagsString=__new0  RConnTagsString=__new0  BranchType=C  Resistance=1.0  Inductance=1.0  SetiL0=off  InitialCurrent=0  Capacitance=1000e-6  Setx0=on  InitialVoltage=700  Measurements=Branch voltage
  C3 : spsSeriesRLCBranchLib/Series RLC Branch  LConnTagsString=__new0  RConnTagsString=__new0  BranchType=C  Resistance=1.0  Inductance=1.0  SetiL0=off  InitialCurrent=0  Capacitance=100e-6  Setx0=on  InitialVoltage=250  Measurements=Branch voltage
  CM2 : spsCurrentMeasurementLib/Current Measurement  Tag=PoWeRsYsTeMmEaSuReMeNt  PhasorSimulation=off  OutputType=Magnitude  PSBequivalent=0
      settings: AttributesFormatString=\n
  Constant : Constant  Value=1000
  Controlled Current Source : spsControlledCurrentSourceLib/Controlled Current Source  Initialize=off  Source_Type=DC  Amplitude=0  Phase=0  Frequency=0  Measurements=None
  Diode1 : spsDiodeLib/Diode  Ron=1e-4  Lon=0  Vf=0  IC=0  UseSnubber=off  Rs=inf  Cs=inf  Measurements=off
  IGBT1 : spsIGBTLib/IGBT  Ron=0.001  Lon=0  Vf=0  Tf=0  Tt=0  IC=0  Rs=1e5  Cs=inf  Measurements=off
  Irradiance Temp1 : Subsystem  Tag=STV Subsys  LoadFcn=sigbuilder_block('load');  StartFcn=sigbuilder_block('start');  StopFcn=sigbuilder_block('stop');  ClipboardFcn=sigbuilder_block('clipboard');  mask(Sigbuilder block){tuvar=[0:10]}
      mask help: Sigbuilder GUI
      mask init:
      | if ~strcmp(get_param(bdroot(gcbh),'SimulationStatus'),'stopped') tuvar = sigbuilder_block('maskInit'); end
      settings: CopyFcn=sigbuilder_block('copy');  DeleteFcn=sigbuilder_block('delete');  ModelCloseFcn=sigbuilder_block('modelClose');  PreSaveFcn=sigbuilder_block('preSave');  PauseFcn=sigbuilder_block('pause')  ContinueFcn=sigbuilder_block('continue')  NameChangeFcn=sigbuilder_block('namechange');  OpenFcn=sigbuilder_block('open',[216.75 153.75 550.5 395.25 ]);  CloseFcn=sigbuilder_block('close');
      mask Display: plot(0, 0, 100, 100,[2, 2, 32, 32, 2], [68, 8, 8, 68, 68],[32, 2], [38, 38], [32, 19, 2],[53, 60, 44], [32, 17, 17, 2],[16, 16, 31, 31]);txt = getActiveGroup(gcbh);text(2, 100, txt,'verticalAlignment', 'top');
  L1 : spsSeriesRLCBranchLib/Series RLC Branch  LConnTagsString=__new0  RConnTagsString=__new0  BranchType=RL  Resistance=0.005  Inductance=5e-3  SetiL0=off  InitialCurrent=0  Capacitance=1e-6  Setx0=off  InitialVoltage=0  Measurements=None
  MPPT : Subsystem
  Memory : Memory  InheritSampleTime=on
  Memory1 : Memory  InheritSampleTime=on
  Memory9 : Memory  InheritSampleTime=on
  Product : Product
  Scope2 : Scope  NumInputPorts=2
  Step1 : Step  Time=5  Before=1000  After=1000  SampleTime=0
  Subsystem1 : Subsystem  mask{A=1.9, T=315, s=1000, Rs=0.01, Rp=400, ns=600, np=3}
      mask prompts: A "Ideality Factor"; T "Surface Temp(K)"; s "Solar Irradiance(W/m^2)"; Rs "Series Resistance"; Rp "Parallel Resistance"; ns "No. of series cell"; np "No. of parallel cell"
      mask init:
      | k=1.38e-23;
      | Voc_n=32.9;
      | Isc_n=10.21;
      | Ki=3.18e-3;
      | Tr=301.15;
      | q=1.6e-19;
      | Eg=1.1;
      | s_n=1000;
  VM1 : spsVoltageMeasurementLib/Voltage Measurement  Tag=PoWeRsYsTeMmEaSuReMeNt  PhasorSimulation=off  OutputType=Magnitude  PSBequivalent=0
  + : PMIOPort  Tag=PMCPort  Side=Right
  _ : PMIOPort  Tag=PMCPort  Port=2  Side=Right
  wires:
  Step1/1 -> Subsystem1/1(s)
  Product/1 -> Scope2/1
  Memory1/1 -> IGBT1/1
  MPPT/1(Out1) -> Memory1/1
  Memory9/1 -> MPPT/2(In2), Product/2
  Memory/1 -> MPPT/1(In1), Product/1
  VM1/1 -> Memory/1, Subsystem1/3(V)
  CM2/1 -> Memory9/1, Subsystem1/2(I)
  Subsystem1/1(I2) -> Controlled Current Source/1
  connections:
  CM2/LConn1 -- Controlled Current Source/RConn1
  L1/LConn1 -- VM1/LConn1 -- CM2/RConn1 -- C3/LConn1
  _/RConn1 -- C1/RConn1 -- IGBT1/RConn1 -- C3/RConn1 -- Controlled Current Source/LConn1 -- VM1/LConn2
  Diode1/LConn1 -- IGBT1/LConn1 -- L1/RConn1
  Diode1/RConn1 -- C1/LConn1 -- +/RConn1

== system Protection/Subsystem ==
  CPL1 : Subsystem
  Ideal Switch2 : spsIdealSwitchLib/Ideal Switch  Ron=0.001  Lon=0  IC=0  Rs=1e5  Cs=inf  Measurements=on
  RL1 : spsSeriesRLCBranchLib/Series RLC Branch  LConnTagsString=__new0  RConnTagsString=__new0  BranchType=R  Resistance=11.52  Inductance=1e-3  SetiL0=off  InitialCurrent=0  Capacitance=5000e-6  Setx0=on  InitialVoltage=1100  Measurements=None
  RL3 : spsSeriesRLCBranchLib/Series RLC Branch  LConnTagsString=__new0  RConnTagsString=__new0  BranchType=R  Resistance=11.52  Inductance=1e-3  SetiL0=off  InitialCurrent=0  Capacitance=5000e-6  Setx0=on  InitialVoltage=1100  Measurements=None
  Step1 : Step  Time=0.5  SampleTime=0
  Step2 : Step  Time=20  SampleTime=0
  + : PMIOPort  Side=Right
  _ : PMIOPort  Port=2  Side=Right
  wires:
  Step2/1 -> Ideal Switch2/1
  connections:
  RL3/RConn1 -- CPL1/RConn2 -- RL1/RConn1
  CPL1/LConn2 -- _/RConn1
  CPL1/LConn1 -- +/RConn1
  RL3/LConn1 -- CPL1/RConn1 -- Ideal Switch2/RConn1
  RL1/LConn1 -- Ideal Switch2/LConn1

== system Protection/Subsystem1 ==
  CPL1 : Subsystem
  Ideal Switch2 : spsIdealSwitchLib/Ideal Switch  Ron=0.001  Lon=0  IC=0  Rs=1e5  Cs=inf  Measurements=on
  RL1 : spsSeriesRLCBranchLib/Series RLC Branch  LConnTagsString=__new0  RConnTagsString=__new0  BranchType=R  Resistance=11.52  Inductance=1e-3  SetiL0=off  InitialCurrent=0  Capacitance=5000e-6  Setx0=on  InitialVoltage=1100  Measurements=None
  RL3 : spsSeriesRLCBranchLib/Series RLC Branch  LConnTagsString=__new0  RConnTagsString=__new0  BranchType=R  Resistance=11.52  Inductance=1e-3  SetiL0=off  InitialCurrent=0  Capacitance=5000e-6  Setx0=on  InitialVoltage=1100  Measurements=None
  Step1 : Step  Time=0.5  SampleTime=0
  Step2 : Step  Time=0  After=0  SampleTime=0
  + : PMIOPort  Side=Right
  _ : PMIOPort  Port=2  Side=Right
  wires:
  Step2/1 -> Ideal Switch2/1
  connections:
  RL3/RConn1 -- CPL1/RConn2 -- RL1/RConn1
  CPL1/LConn2 -- _/RConn1
  CPL1/LConn1 -- +/RConn1
  RL3/LConn1 -- CPL1/RConn1 -- Ideal Switch2/RConn1
  RL1/LConn1 -- Ideal Switch2/LConn1

== system Protection/Subsystem10 ==
  note: Reference:
      | V. Nougain, S. Mishra, G. S. Misyris and S. Chatzivasileiadis, "Multiterminal DC Fault Identification for MMC-HVDC Systems Based on Modal Analysis—A Localized Protection Scheme," in IEEE Journal of Emerging and Selected Topics in Power Electronics , vol. 9, no. 6, pp. 6650-6661, Dec. 2021, doi: 10.1109/JESTPE.2021.3068800.
  Scope1 : Scope  NumInputPorts=4
  Subtract{,1..3} (4 alike) : Sum  Inputs=+-
  tag scope: U1=global, U2=global
  wires:
  [Vdc2] -> Subtract1/2
  Subtract3/1 -> Scope1/4
  [V6] -> Subtract3/1
  [Vdc3] -> Subtract2/2
  [V3] -> Subtract2/1
  [Udc1] -> Subtract/2
  Subtract2/1 -> Scope1/3
  [V2] -> Subtract1/1
  Subtract/1 -> [U1], Scope1/1
  Subtract1/1 -> [U2], Scope1/2
  [V1] -> Subtract/1
  [Vdc6] -> Subtract3/2

== system Protection/Subsystem2 ==
  Breaker2 : spsBreakerLib/Breaker  InitialState=0  SwitchingTimes="[1.04  1.5]"  External=off  BreakerResistance=0.01  SnubberResistance=1e6  SnubberCapacitance=inf  Measurements=None  MoreParameters=on  NoBreakLoop=off
  Conn1 : PMIOPort  Side=Right
  Conn2 : PMIOPort  Port=2  Side=Left
  connections:
  Breaker2/RConn1 -- Conn2/RConn1
  Breaker2/LConn1 -- Conn1/RConn1

== system Protection/Subsystem3 ==
  Breaker2 : spsBreakerLib/Breaker  InitialState=0  SwitchingTimes="[1.04  1.5]"  External=off  BreakerResistance=0.01  SnubberResistance=1e6  SnubberCapacitance=inf  Measurements=None  MoreParameters=on  NoBreakLoop=off
  Conn1 : PMIOPort  Side=Right
  Conn2 : PMIOPort  Port=2  Side=Left
  connections:
  Breaker2/RConn1 -- Conn2/RConn1
  Breaker2/LConn1 -- Conn1/RConn1

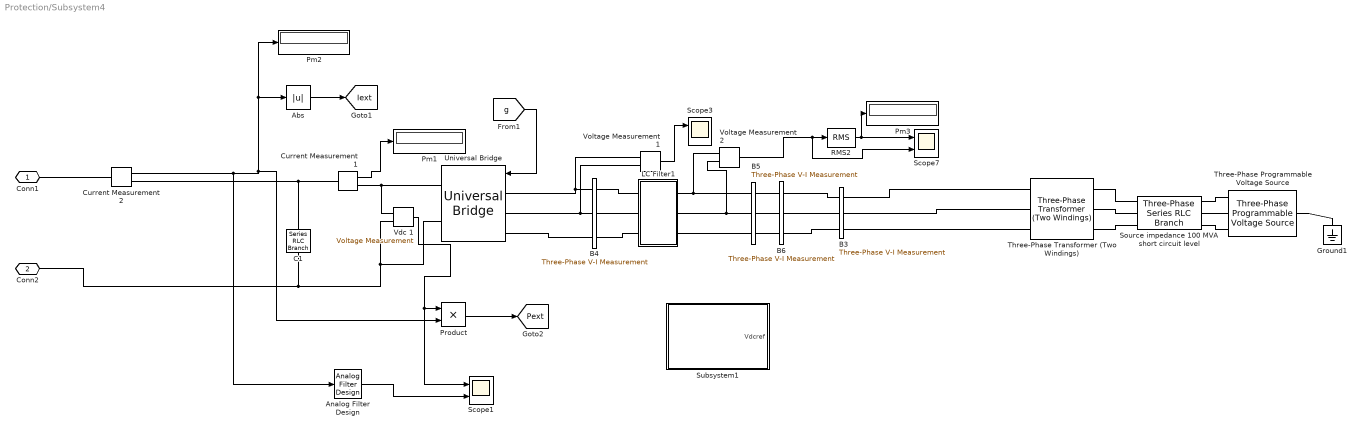
== system Protection/Subsystem4 ==
  Abs : Abs  SaturateOnIntegerOverflow=off
  Analog Filter Design : dspfdesign/Analog Filter Design  method=Butterworth  filttype=Lowpass  N=1  Wlo=30  Whi=80  Rp=2  Rs=40
  B3 : spsThreePhaseVIMeasurementLib/Three-Phase V-I Measurement  VoltageMeasurement=phase-to-ground  SetLabelV=on  LabelV=Vb1  Vpu=off  VpuLL=off  CurrentMeasurement=yes  SetLabelI=on  LabelI=Ib1  Ipu=off  Pbase=100e6  Vbase=735e3  OutputType=Complex  PhasorSimulation=off  PSBequivalent=0
  B4 : spsThreePhaseVIMeasurementLib/Three-Phase V-I Measurement  VoltageMeasurement=no  SetLabelV=off  LabelV=Vabc_B1  Vpu=off  VpuLL=off  CurrentMeasurement=yes  SetLabelI=on  LabelI=IL  Ipu=off  Pbase=100e6  Vbase=735e3  OutputType=Complex  PhasorSimulation=off  PSBequivalent=0
  B5 : spsThreePhaseVIMeasurementLib/Three-Phase V-I Measurement  VoltageMeasurement=phase-to-ground  SetLabelV=on  LabelV=Vo  Vpu=off  VpuLL=off  CurrentMeasurement=yes  SetLabelI=on  LabelI=Io  Ipu=off  Pbase=100e6  Vbase=735e3  OutputType=Complex  PhasorSimulation=off  PSBequivalent=0
  B6 : spsThreePhaseVIMeasurementLib/Three-Phase V-I Measurement  VoltageMeasurement=phase-to-ground  SetLabelV=on  LabelV=Vabcg  Vpu=on  VpuLL=off  CurrentMeasurement=yes  SetLabelI=on  LabelI=Iabcg  Ipu=off  Pbase=100e3  Vbase=415  OutputType=Magnitude  PhasorSimulation=off  PSBequivalent=0
  C1 : spsSeriesRLCBranchLib/Series RLC Branch  LConnTagsString=__new0  RConnTagsString=__new0  BranchType=C  Resistance=1.0  Inductance=1.0  SetiL0=off  InitialCurrent=0  Capacitance=5000e-6  Setx0=on  InitialVoltage=700  Measurements=Branch voltage
  Current Measurement1 : spsCurrentMeasurementLib/Current Measurement  PhasorSimulation=off  OutputType=Complex  PSBequivalent=0
  Current Measurement2 : spsCurrentMeasurementLib/Current Measurement  PhasorSimulation=off  OutputType=Complex  PSBequivalent=0
  Ground1 : spsGroundLib/Ground  LConnTagsString=a
  LC Filter1 : Subsystem
  Pm1 : Display
  Pm2 : Display
  Pm3 : Display
  Product : Product
  RMS2 : powerlib_extras/Measurements/RMS  f1=50
  Scope1 : Scope  NumInputPorts=2
  Scope3 : Scope  NumInputPorts=2
  Scope7 : Scope  NumInputPorts=2
  Source impedance 100 MVA short circuit level : spsThreePhaseSeriesRLCBranchLib/Three-Phase Series RLC Branch  LConnTagsString=A|B|C  RConnTagsString=A|B|C  BranchType=RL  Resistance=11^2/1000/5  Inductance=11^2/1000/(2*pi*50)  Capacitance=1.0  Measurements=None
  Subsystem1 : Subsystem
  Three-Phase Programmable Voltage Source : spsThreePhaseProgrammableVoltageSourceLib/Three-Phase Programmable Voltage Source  PositiveSequence="[11000  0 50]"  VariationEntity=None  VariationType=Table of time-amplitude pairs  VariationTypeAlt=Step  VariationStep=0.5  VariationRate=10  VariationMagnitude=0.3  VariationFrequency=2  VariationTiming=[1 2]  VariationPhaseA=off  Amplitudes=[1 0.8 1.2 1.0]  TimeValues=[0 0.1 0.15 0.2]  HarmonicGeneration=off  HarmonicA=[3 0.2 -25 0]  HarmonicB=[2 0.15 35 2]  Timing="[0.05  3]"  BusType=swing  Pref=0  Qref=0  Qmin=-inf  Qmax=inf
  Three-Phase Transformer (Two Windings) : spsThreePhaseTransformerTwoWindingsLib/Three-Phase Transformer (Two Windings)  Winding1Connection=Yg  Winding2Connection=Delta (D1)  CoreType=Three single-phase transformers  SetSaturation=off  Hysteresis=off  DataFile='hysteresis'  SetInitialFlux=off  Measurements=None  UNITS=pu  NominalPower=[ 50e3 , 50 ]  Winding1=[ 0.415e3 , 0.002 , 0.08 ]  Winding2=[ 11e3 , 0.002 , 0.08 ]  Rm=500  Lm=500  L0=0.5  Saturation=[ 0,0 ; 0.0024,1.2 ; 1.0,1.52 ]  InitialFluxes=[ 0.8 , -0.8 , 0.7 ]  BreakLoop=off  DiscreteSolver=Trapezoidal iterative  DataType=off  TransfoNumber=1
  Universal Bridge : spsUniversalBridgeLib/Universal Bridge  Arms=3  SnubberResistance=5000  SnubberCapacitance=inf  Device=IGBT / Diodes  Ron=3e-3  Lon=0  ForwardVoltages="[  0  0  ]"  ForwardVoltage=0  GTOparameters=[ 1e-6 , 2e-6 ]  IGBTparameters=[ 1e-6 , 2e-6 ]  Measurements=All voltages and currents  Measurements_2=None  converterType=Rectifier
  Vdc 1 : spsVoltageMeasurementLib/Voltage Measurement  Tag=PoWeRsYsTeMmEaSuReMeNt  PhasorSimulation=off  OutputType=Magnitude  PSBequivalent=0
  Voltage Measurement1 : spsVoltageMeasurementLib/Voltage Measurement  PhasorSimulation=off  OutputType=Complex  PSBequivalent=0
  Voltage Measurement2 : spsVoltageMeasurementLib/Voltage Measurement  PhasorSimulation=off  OutputType=Complex  PSBequivalent=0
  Conn1 : PMIOPort  Side=Left
  Conn2 : PMIOPort  Port=2  Side=Left
  tag scope: Iext=global, Pext=global
  wires:
  Voltage Measurement2/1 -> Scope7/2, RMS2/1
  Voltage Measurement1/1 -> Scope3/1
  [g] -> Universal Bridge/1
  Current Measurement1/1 -> Pm1/1
  Product/1 -> [Pext]
  RMS2/1 -> Pm3/1, Scope7/1
  ? -> Scope3/2
  Abs/1 -> [Iext]
  Current Measurement2/1 -> Analog Filter Design/1, Product/2, Abs/1, Pm2/1
  Vdc 1/1 -> Scope1/1, Product/1
  Analog Filter Design/1 -> Scope1/2
  connections:
  B5/RConn2 -- B6/LConn2
  Vdc 1/LConn2 -- Conn2/RConn1 -- C1/RConn1 -- Universal Bridge/RConn2
  B3/LConn2 -- B6/RConn2
  B6/RConn3 -- B3/LConn3
  B4/RConn1 -- LC Filter1/LConn1
  B5/RConn3 -- B6/LConn3
  B6/RConn1 -- B3/LConn1
  LC Filter1/RConn2 -- Voltage Measurement2/LConn2 -- B5/LConn2
  B4/RConn3 -- LC Filter1/LConn3
  B5/LConn3 -- LC Filter1/RConn3
  LC Filter1/RConn1 -- Voltage Measurement2/LConn1 -- B5/LConn1
  B4/LConn1 -- Universal Bridge/LConn1 -- Voltage Measurement1/LConn1
  Current Measurement1/RConn1 -- Universal Bridge/RConn1 -- Vdc 1/LConn1
  B4/LConn2 -- Universal Bridge/LConn2 -- Voltage Measurement1/LConn2
  Current Measurement2/LConn1 -- Conn1/RConn1
  B5/RConn1 -- B6/LConn1
  B4/RConn2 -- LC Filter1/LConn2
  Three-Phase Transformer (Two Windings)/LConn1 -- B3/RConn1
  Three-Phase Transformer (Two Windings)/LConn2 -- B3/RConn2
  Three-Phase Transformer (Two Windings)/LConn3 -- B3/RConn3
  B4/LConn3 -- Universal Bridge/LConn3
  Three-Phase Programmable Voltage Source/LConn1 -- Ground1/LConn1
  Source impedance 100 MVA short circuit level/RConn1 -- Three-Phase Programmable Voltage Source/RConn1
  Source impedance 100 MVA short circuit level/RConn2 -- Three-Phase Programmable Voltage Source/RConn2
  Source impedance 100 MVA short circuit level/RConn3 -- Three-Phase Programmable Voltage Source/RConn3
  Three-Phase Transformer (Two Windings)/RConn1 -- Source impedance 100 MVA short circuit level/LConn1
  Source impedance 100 MVA short circuit level/LConn2 -- Three-Phase Transformer (Two Windings)/RConn2
  Three-Phase Transformer (Two Windings)/RConn3 -- Source impedance 100 MVA short circuit level/LConn3
  Current Measurement2/RConn1 -- Current Measurement1/LConn1 -- C1/LConn1

== system Protection/Subsystem5 ==
  Breaker2 : spsBreakerLib/Breaker  InitialState=0  SwitchingTimes=[1.04]  External=off  BreakerResistance=0.01  SnubberResistance=1e6  SnubberCapacitance=inf  Measurements=None  MoreParameters=on  NoBreakLoop=off
  Conn1 : PMIOPort  Side=Right
  Conn2 : PMIOPort  Port=2  Side=Left
  connections:
  Breaker2/RConn1 -- Conn2/RConn1
  Breaker2/LConn1 -- Conn1/RConn1

== system Protection/Subsystem6 ==
  Breaker2 : spsBreakerLib/Breaker  InitialState=0  SwitchingTimes="[1.04  1.5]"  External=off  BreakerResistance=0.01  SnubberResistance=1e6  SnubberCapacitance=inf  Measurements=None  MoreParameters=on  NoBreakLoop=off
  Conn1 : PMIOPort  Side=Right
  Conn2 : PMIOPort  Port=2  Side=Left
  connections:
  Breaker2/RConn1 -- Conn2/RConn1
  Breaker2/LConn1 -- Conn1/RConn1

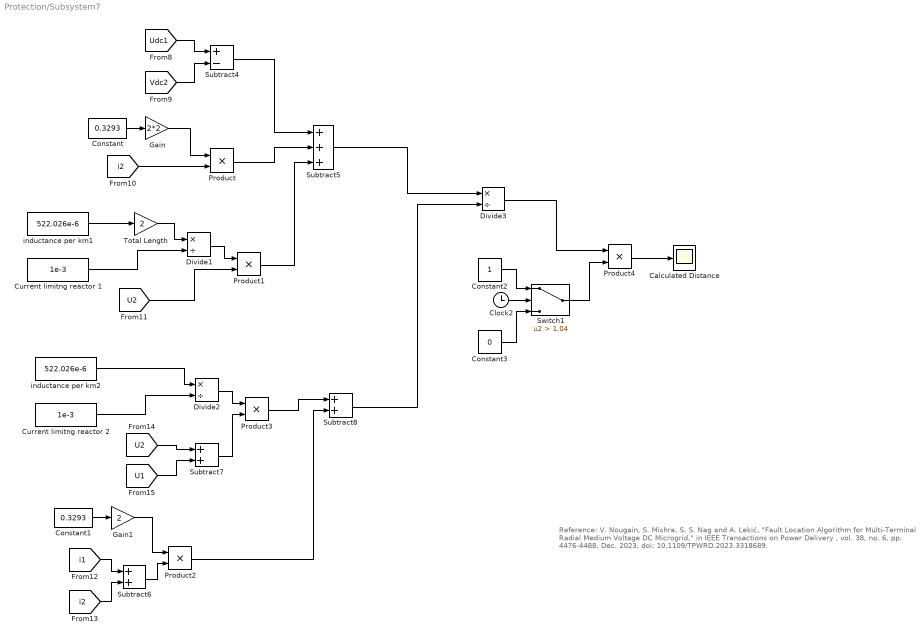
== system Protection/Subsystem7 ==
  note: Reference:
      | V. Nougain, S. Mishra, S. S. Nag and A. Lekić, "Fault Location Algorithm for Multi-Terminal Radial Medium Voltage DC Microgrid," in IEEE Transactions on Power Delivery , vol. 38, no. 6, pp. 4476-4488, Dec. 2023, doi: 10.1109/TPWRD.2023.3318689.
  Calculated Distance : Scope
  Clock2 : Clock
      settings: Decimation=6
  Constant : Constant  Value=0.3293
  Constant1 : Constant  Value=0.3293
  Constant2 : Constant
  Constant3 : Constant  Value=0
  Current limitng reactor 1 : Constant  Value=1e-3
  Current limitng reactor 2 : Constant  Value=1e-3
  Divide1 : Product  Inputs=*/
  Divide2 : Product  Inputs=*/
  Divide3 : Product  Inputs=*/
  Gain : Gain  Gain=2*2
  Gain1 : Gain  Gain=2
  Product{,1..4} (5 alike) : Product
  Subtract4 : Sum  Inputs=+-
  Subtract5 : Sum  Inputs=+++
  Subtract6 : Sum
  Subtract7 : Sum
  Subtract8 : Sum
  Switch1 : Switch  Criteria=u2 > Threshold  Threshold=1.04  SaturateOnIntegerOverflow=off  InputSameDT=off
  Total Length : Gain  Gain=2
  inductance per km1 : Constant  Value=522.026e-6
  inductance per km2 : Constant  Value=522.026e-6
  wires:
  [Udc1] -> Subtract4/1
  Product/1 -> Subtract5/2
  Product1/1 -> Subtract5/3
  Current limitng reactor 2/1 -> Divide2/2
  Subtract6/1 -> Product2/2
  Divide1/1 -> Product1/1
  inductance per km1/1 -> Total Length/1
  Subtract7/1 -> Product3/2
  Total Length/1 -> Divide1/1
  Current limitng reactor 1/1 -> Divide1/2
  [i1] -> Subtract6/1
  [U2] -> Product1/2
  Product2/1 -> Subtract8/2
  Product3/1 -> Subtract8/1
  [Vdc2] -> Subtract4/2
  Subtract5/1 -> Divide3/1
  Subtract4/1 -> Subtract5/1
  [U2] -> Subtract7/1
  Gain1/1 -> Product2/1
  Divide2/1 -> Product3/1
  Constant/1 -> Gain/1
  [i2] -> Subtract6/2
  Constant1/1 -> Gain1/1
  [U1] -> Subtract7/2
  Subtract8/1 -> Divide3/2
  Gain/1 -> Product/1
  inductance per km2/1 -> Divide2/1
  [i2] -> Product/2
  Divide3/1 -> Product4/1
  Constant2/1 -> Switch1/1
  Clock2/1 -> Switch1/2
  Constant3/1 -> Switch1/3
  Switch1/1 -> Product4/2
  Product4/1 -> Calculated Distance/1

== system Protection/Subsystem8 ==
  Breaker2 : spsBreakerLib/Breaker  InitialState=0  SwitchingTimes="[1.04  1.5]"  External=off  BreakerResistance=0.01  SnubberResistance=1e6  SnubberCapacitance=inf  Measurements=None  MoreParameters=on  NoBreakLoop=off
  Conn1 : PMIOPort  Side=Right
  Conn2 : PMIOPort  Port=2  Side=Left
  connections:
  Breaker2/RConn1 -- Conn2/RConn1
  Breaker2/LConn1 -- Conn1/RConn1

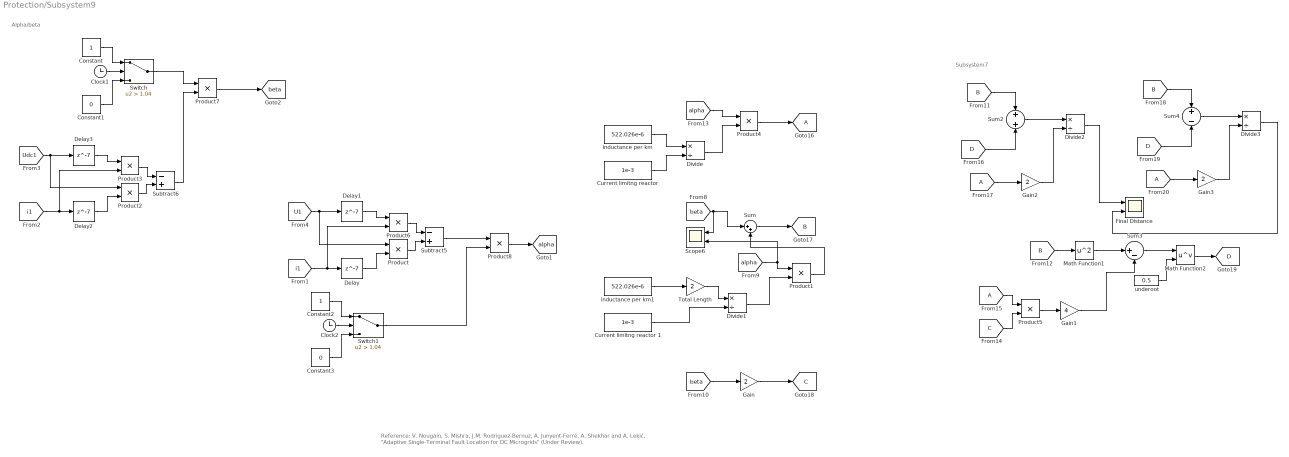
== system Protection/Subsystem9 ==
  note: Alpha/beta
  note: Subsystem7
  note: Reference:
      | V. Nougain, S. Mishra, J.M. Rodriguez-Bernuz, A. Junyent-Ferré, A. Shekhar and A. Lekić, "Adaptive Single-Terminal Fault Location for DC Microgrids" (Under Review).
  Clock1 : Clock
      settings: Decimation=6
  Clock2 : Clock
      settings: Decimation=6
  Constant : Constant
  Constant1 : Constant  Value=0
  Constant2 : Constant
  Constant3 : Constant  Value=0
  "Current limitng reactor " : Constant  Value=1e-3
  Current limitng reactor 1 : Constant  Value=1e-3
  Delay{,1..3} (4 alike) : Delay  DelayLength=7  InitialCondition=0
  Divide{,1..3} (4 alike) : Product  Inputs=*/
  Final Distance : Scope  NumInputPorts=2
  From15 : From  TagVisibility=global
  From17 : From  TagVisibility=global
  From20 : From  TagVisibility=global
  Gain : Gain  Gain=2
  Gain1 : Gain  Gain=4
  Gain2 : Gain  Gain=2
  Gain3 : Gain  Gain=2
  Goto16 : Goto  TagVisibility=global
  Math Function1 : Math  Operator=square
  Math Function2 : Math  Operator=pow
  Product{,1..8} (9 alike) : Product
  Scope6 : Scope  NumInputPorts=2
  Subtract5 : Sum  Inputs=-+
  Subtract6 : Sum  Inputs=-+
  Sum : Sum  Inputs=|++
  Sum2 : Sum
  Sum3 : Sum  Inputs=|+-
  Sum4 : Sum  Inputs=+-
  Switch : Switch  Criteria=u2 > Threshold  Threshold=1.04  SaturateOnIntegerOverflow=off  InputSameDT=off
  Switch1 : Switch  Criteria=u2 > Threshold  Threshold=1.04  SaturateOnIntegerOverflow=off  InputSameDT=off
  Total Length : Gain  Gain=2
  inductance per km : Constant  Value=522.026e-6
  inductance per km1 : Constant  Value=522.026e-6
  underoot : Constant  Value=0.5
  tag scope: B=global, C=global, D=global, alpha=global, beta=global
  wires:
  Product4/1 -> Goto16/1
  Current limitng reactor 1/1 -> Divide1/2
  Sum/1 -> [B]
  inductance per km/1 -> Divide/1
  [alpha] -> Product4/1
  Divide/1 -> Product4/2
  [beta] -> Scope6/1, Sum/1
  [beta] -> Gain/1
  [alpha] -> Product1/1, Scope6/2
  Divide1/1 -> Product1/2
  "Current limitng reactor "/1 -> Divide/2
  Product1/1 -> Sum/2
  inductance per km1/1 -> Total Length/1
  Total Length/1 -> Divide1/1
  Gain/1 -> [C]
  Divide3/1 -> Final Distance/2
  [B] -> Sum2/1
  Sum4/1 -> Divide3/1
  [D] -> Sum4/2
  Divide2/1 -> Final Distance/1
  Gain1/1 -> Sum3/2
  Gain3/1 -> Divide3/2
  Math Function1/1 -> Sum3/1
  From17/1 -> Gain2/1
  [B] -> Sum4/1
  underoot/1 -> Math Function2/2
  Sum2/1 -> Divide2/1
  Math Function2/1 -> [D]
  From20/1 -> Gain3/1
  [B] -> Math Function1/1
  Sum3/1 -> Math Function2/1
  [C] -> Product5/2
  Gain2/1 -> Divide2/2
  From15/1 -> Product5/1
  [D] -> Sum2/2
  Product5/1 -> Gain1/1
  Product8/1 -> [alpha]
  Constant3/1 -> Switch1/3
  Constant2/1 -> Switch1/1
  Clock2/1 -> Switch1/2
  Switch1/1 -> Product8/2
  Subtract5/1 -> Product8/1
  Product7/1 -> [beta]
  Subtract6/1 -> Product7/2
  Switch/1 -> Product7/1
  Constant1/1 -> Switch/3
  Constant/1 -> Switch/1
  Clock1/1 -> Switch/2
  Product6/1 -> Subtract5/1
  Product/1 -> Subtract5/2
  Delay2/1 -> Product2/2
  Product3/1 -> Subtract6/1
  Product2/1 -> Subtract6/2
  Delay3/1 -> Product3/1
  Delay1/1 -> Product6/1
  [i1] -> Product6/2, Delay/1
  [i1] -> Product3/2, Delay2/1
  [U1] -> Product/1, Delay1/1
  [Udc1] -> Product2/1, Delay3/1
  Delay/1 -> Product/2

== system Protection/PV /Irradiance Temp1 ==
  Demux : Demux  Tag=STV Demux  Outputs=2
      settings: DisplayOption=none
  FromWs : FromWorkspace  Tag=STV FromWs  VariableName=tuvar
      SigBuilderData=|
      | common.afterFinalStr = 'Extrapolate'
      | common.sampleTime = '0'
      | dataSet(1).timeRange = [0 1]
      | dataSet(1).name = 'Constant Irradiance'
      | dataSet(2).timeRange = [0 1]
      | dataSet(2).name = 'Step Irradiance'
      | dataSet(3).timeRange = [0 10]
      | dataSet(3).name = 'Ramp-up/down Irradiance'
      | sbobj.Groups(1).Name = 'Constant Irradiance'
      | sbobj.Groups(1).Signals(1).Name = 'Ir'
      | sbobj.Groups(1).Signals(1).XData = [0 1]
      | sbobj.Groups(1).Signals(1).YData = [1000 1000]
      | sbobj.Groups(1).Signals(2).Name = 'Temp'
      | sbobj.Groups(1).Signals(2).XData = [0 1 1 2]
      | sbobj.Groups(1).Signals(2).YData = [0 0 1 1]
      | sbobj.Groups(1).TimeRange = [0 1]
      | sbobj.Groups(2).Name = 'Step Irradiance'
      | sbobj.Groups(2).Signals(1).Name = 'Ir'
      | sbobj.Groups(2).Signals(1).XData = [0 0.252 0.252 1]
      | sbobj.Groups(2).Signals(1).YData = [600 600 1000 1000]
      | sbobj.Groups(2).Signals(2).Name = 'Temp'
      | sbobj.Groups(2).Signals(2).XData = [0 1 1 2]
      | sbobj.Groups(2).Signals(2).YData = [0 0 1 1]
      | sbobj.Groups(2).TimeRange = [0 1]
      | sbobj.Groups(3).Name = 'Ramp-up/down Irradiance'
      | sbobj.Groups(3).Signals(1).Name = 'Ir'
      | sbobj.Groups(3).Signals(1).XData = [0 3 4 6 7 10]
      | sbobj.Groups(3).Signals(1).YData = [1000 1000 500 500 800 800]
      | sbobj.Groups(3).Signals(2).Name = 'Temp'
      | sbobj.Groups(3).Signals(2).XData = [0 2 2.1 10]
      | sbobj.Groups(3).Signals(2).YData = [25 25 25 25]
  Ir : Outport  Tag=STV Outport
  Temp : Outport  Tag=STV Outport  Port=2
  wires:
  Demux/1 -> Ir/1
  FromWs/1 -> Demux/1
  Demux/2 -> Temp/1

== system Protection/PV /MPPT ==
  In1 : Inport
  In2 : Inport  Port=2
  Add1 : Sum  Inputs=-+
  Constant1 : Constant  Value=0
  Constant2 : Constant  Value=0.5
  Constant3 : Constant
  MPPT : Subsystem
  Relational Operator : RelationalOperator  Operator=<  OutDataTypeStr=boolean  InputSameDT=off
  Repeating Sequence : simulink/Sources/Repeating Sequence  rep_seq_t=[0 0.00005 0.0001]  rep_seq_y=[0 1 0]
  Sign : Signum
  Switch2 : Switch  Criteria=u2 > Threshold  SaturateOnIntegerOverflow=off  InputSameDT=off
  Unit Delay1 : UnitDelay  SampleTime=2e-6  HasFrameUpgradeWarning=on
  Unit Delay2 : UnitDelay  SampleTime=2e-6  HasFrameUpgradeWarning=on
  Out1 : Outport
  wires:
  MPPT/1(sign) -> Sign/1
  Unit Delay1/1 -> MPPT/1(V_PV)
  Unit Delay2/1 -> MPPT/2(I_PV)
  Constant1/1 -> Switch2/1
  Sign/1 -> Switch2/2
  Constant3/1 -> Switch2/3
  Switch2/1 -> Add1/1
  In1/1 -> Unit Delay1/1
  In2/1 -> Unit Delay2/1
  Constant2/1 -> Add1/2
  Add1/1 -> Relational Operator/1
  Repeating Sequence/1 -> Relational Operator/2
  Relational Operator/1 -> Out1/1

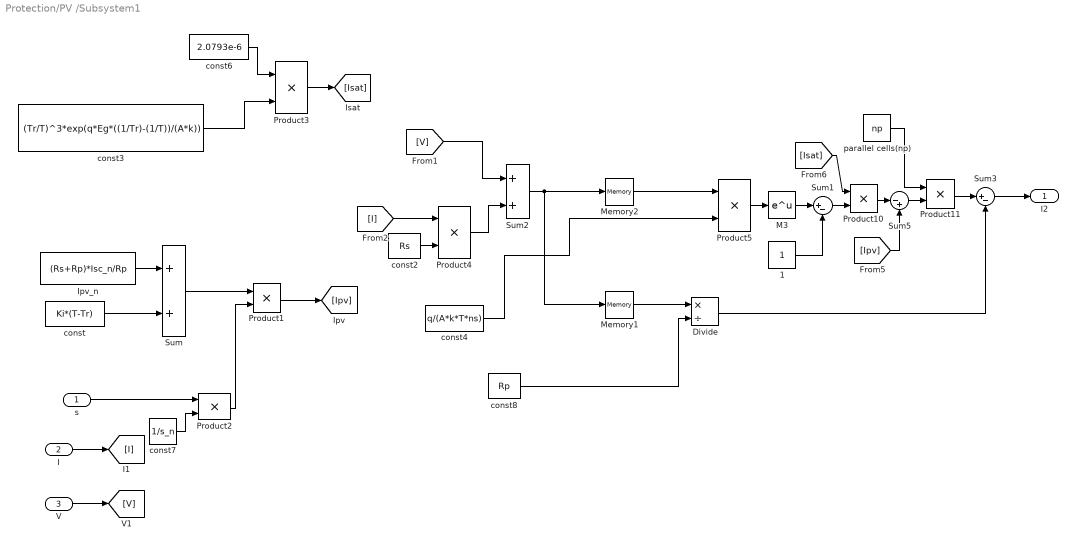
== system Protection/PV /Subsystem1 ==
  s : Inport
  I : Inport  Port=2
  V : Inport  Port=3
  1 : Constant
  Divide : Product  Inputs=*/
  Ipv_n : Constant  Value=(Rs+Rp)*Isc_n/Rp
  M3 : Math  SignedPower=on
  Memory1 : Memory
  Memory2 : Memory
  Product{1..5,10..11} (7 alike) : Product  RndMeth=Zero
  Sum : Sum
  Sum1 : Sum  Inputs=|+-
  Sum2 : Sum
  Sum3 : Sum  Inputs=|+-
  Sum5 : Sum  Inputs=|-+
  const : Constant  Value=Ki*(T-Tr)
  const2 : Constant  Value=Rs
  const3 : Constant  Value=(Tr/T)^3*exp(q*Eg*((1/Tr)-(1/T))/(A*k))
  const4 : Constant  Value=q/(A*k*T*ns)
  const6 : Constant  Value=2.0793e-6
  const7 : Constant  Value=1/s_n
  const8 : Constant  Value=Rp
  parallel cells(np) : Constant  Value=np
  I2 : Outport
  wires:
  const6/1 -> Product3/1
  const/1 -> Sum/2
  Sum/1 -> Product1/1
  Product1/1 -> [Ipv]
  const3/1 -> Product3/2
  Product3/1 -> [Isat]
  V/1 -> [V]
  I/1 -> [I]
  [V] -> Sum2/1
  const2/1 -> Product4/2
  [I] -> Product4/1
  const4/1 -> Product5/2
  Product5/1 -> M3/1
  M3/1 -> Sum1/1
  1/1 -> Sum1/2
  Sum1/1 -> Product10/2
  [Isat] -> Product10/1
  [Ipv] -> Sum5/2
  Product10/1 -> Sum5/1
  Sum5/1 -> Product11/2
  parallel cells(np)/1 -> Product11/1
  Sum2/1 -> Memory2/1, Memory1/1
  Product2/1 -> Product1/2
  s/1 -> Product2/1
  const7/1 -> Product2/2
  Product4/1 -> Sum2/2
  Ipv_n/1 -> Sum/1
  const8/1 -> Divide/2
  Product11/1 -> Sum3/1
  Sum3/1 -> I2/1
  Divide/1 -> Sum3/2
  Memory1/1 -> Divide/1
  Memory2/1 -> Product5/1

== system Protection/PV 1/Irradiance Temp1 ==
  Demux : Demux  Tag=STV Demux  Outputs=2
      settings: DisplayOption=none
  FromWs : FromWorkspace  Tag=STV FromWs  VariableName=tuvar
      SigBuilderData=|
      | common.afterFinalStr = 'Extrapolate'
      | common.sampleTime = '0'
      | dataSet(1).timeRange = [0 1]
      | dataSet(1).name = 'Constant Irradiance'
      | dataSet(2).timeRange = [0 1]
      | dataSet(2).name = 'Step Irradiance'
      | dataSet(3).timeRange = [0 10]
      | dataSet(3).name = 'Ramp-up/down Irradiance'
      | sbobj.Groups(1).Name = 'Constant Irradiance'
      | sbobj.Groups(1).Signals(1).Name = 'Ir'
      | sbobj.Groups(1).Signals(1).XData = [0 1]
      | sbobj.Groups(1).Signals(1).YData = [1000 1000]
      | sbobj.Groups(1).Signals(2).Name = 'Temp'
      | sbobj.Groups(1).Signals(2).XData = [0 1 1 2]
      | sbobj.Groups(1).Signals(2).YData = [0 0 1 1]
      | sbobj.Groups(1).TimeRange = [0 1]
      | sbobj.Groups(2).Name = 'Step Irradiance'
      | sbobj.Groups(2).Signals(1).Name = 'Ir'
      | sbobj.Groups(2).Signals(1).XData = [0 0.252 0.252 1]
      | sbobj.Groups(2).Signals(1).YData = [600 600 1000 1000]
      | sbobj.Groups(2).Signals(2).Name = 'Temp'
      | sbobj.Groups(2).Signals(2).XData = [0 1 1 2]
      | sbobj.Groups(2).Signals(2).YData = [0 0 1 1]
      | sbobj.Groups(2).TimeRange = [0 1]
      | sbobj.Groups(3).Name = 'Ramp-up/down Irradiance'
      | sbobj.Groups(3).Signals(1).Name = 'Ir'
      | sbobj.Groups(3).Signals(1).XData = [0 3 4 6 7 10]
      | sbobj.Groups(3).Signals(1).YData = [1000 1000 500 500 800 800]
      | sbobj.Groups(3).Signals(2).Name = 'Temp'
      | sbobj.Groups(3).Signals(2).XData = [0 2 2.1 10]
      | sbobj.Groups(3).Signals(2).YData = [25 25 25 25]
  Ir : Outport  Tag=STV Outport
  Temp : Outport  Tag=STV Outport  Port=2
  wires:
  Demux/2 -> Temp/1
  FromWs/1 -> Demux/1
  Demux/1 -> Ir/1
